simulink model "simulatore_motore"  (Simulink 8.3)
settings: Solver=ode45  StartTime=0.0  StopTime=30  RelTol=1e-3
values from neighbouring files (symbols this model uses):
  Beta = 17.7e-6    (= 1.77e-05)    [es1.m]
  J = 19.74e-6    (= 1.974e-05)    [es1.m]
  Km = 0.0535    [es1.m]
  Kpwm = 2.925    [es1.m]
  Kt = 0.02    [es1.m]
  La = 3.24e-3    (= 0.00324)    [es1.m]
  Ra = 6    [es1.m]
  Rs = 7.525    [es1.m]
  s = tf('s')    [es1.m]
  tau_a = 0.001    [es1.m]
  Td = -1e-4    (= -0.0001)    [es1.m]
libraries: cstblocks x8
settings Model: Creator=Indri  LastModifiedBy=HP  ExtModeTrigMode=oneshot  ExtModeArmWhenConnect=off
settings DataIOCC: LimitDataPoints=off
settings OptimizationCC: BlockReduction=off  BooleanDataType=off  ExpressionDepthLimit=2147483647  InitFltsAndDblsToZero=on
settings DebuggingCC: SaveWithParameterizedLinksMsg=none  SignalResolutionControl=TryResolveAllWithWarning  SolverPrmCheckMsg=none  MultiTaskDSMMsg=warning  MultiTaskCondExecSysMsg=none  FcnCallInpInsideContextMsg=UseLocalSettings
settings HardwareCC: TargetUnknown=on
settings RTWCC: IncludeERTFirstTime=on
settings GRTTargetCC: TargetFcnLib=ansi_tfl_tmw.mat

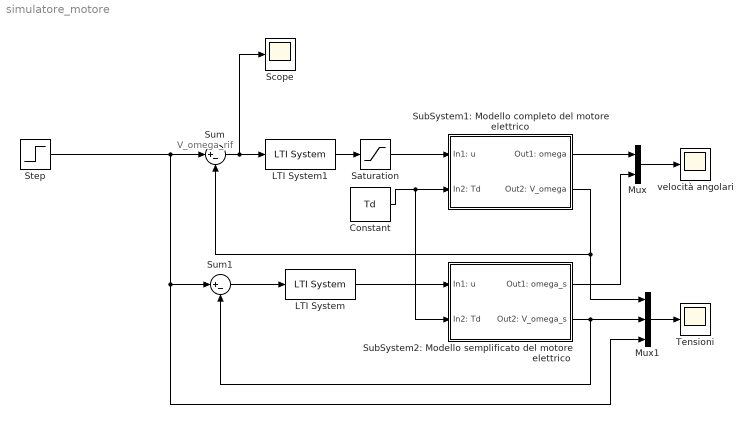
== system simulatore_motore ==
  note: V_omega_rif
  Constant : Constant  Value=Td
  LTI System : cstblocks/LTI System  sys=Cd  IC=[]
  LTI System1 : cstblocks/LTI System  sys=Cd  IC=[]
  Mux : Mux  Inputs=2
  Mux1 : Mux  Inputs=3
  Saturation : Saturate  UpperLimit=5  LowerLimit=-5
  Scope : Scope
      settings: MaxDataPoints=50000
  Step : Step  SampleTime=0
  SubSystem1: Modello completo del motore elettrico : Subsystem
  SubSystem2: Modello semplificato del motore elettrico : Subsystem
  Sum : Sum  Inputs=|+-  SaturateOnIntegerOverflow=on  InputSameDT=on  OutDataTypeStr=Inherit: Same as first input
  Sum1 : Sum  Inputs=|+-  SaturateOnIntegerOverflow=on  InputSameDT=on  OutDataTypeStr=Inherit: Same as first input
  Tensioni : Scope
      settings: YMin=-0.05  YMax=1
  velocità angolari : Scope
      settings: YMin=-2.5  YMax=50
  wires:
  SubSystem2: Modello semplificato del motore elettrico/1(Out1: omega_s) -> Mux/2
  SubSystem1: Modello completo del motore elettrico/1(Out1: omega) -> Mux/1
  Mux/1 -> velocità angolari/1
  Step/1 -> Sum/1, Sum1/1, Mux1/3
  Constant/1 -> SubSystem1: Modello completo del motore elettrico/2(In2: Td), SubSystem2: Modello semplificato del motore elettrico/2(In2: Td)
  SubSystem2: Modello semplificato del motore elettrico/2(Out2: V_omega_s) -> Sum1/2, Mux1/2
  Mux1/1 -> Tensioni/1
  SubSystem1: Modello completo del motore elettrico/2(Out2: V_omega) -> Sum/2, Mux1/1
  Sum1/1 -> LTI System/1
  LTI System/1 -> SubSystem2: Modello semplificato del motore elettrico/1(In1: u)
  Sum/1 -> Scope/1, LTI System1/1
  LTI System1/1 -> Saturation/1
  Saturation/1 -> SubSystem1: Modello completo del motore elettrico/1(In1: u)

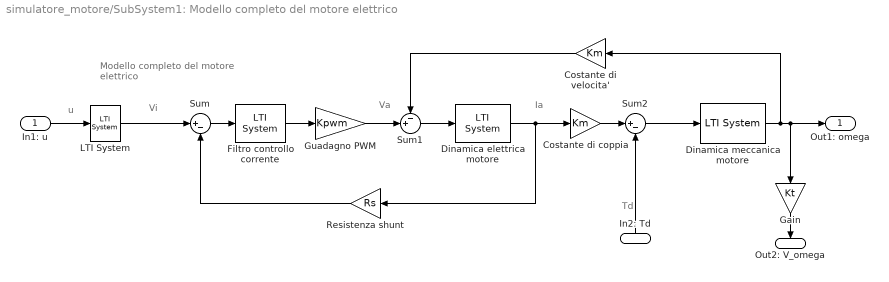
== system simulatore_motore/SubSystem1: Modello completo del motore elettrico ==
  note: Vi
  note: Ia
  note: Va
  note: u
  note: Td
  note: Modello completo
      | del motore elettrico
  In1: u : Inport
  In2: Td : Inport  Port=2
  Costante di coppia : Gain  Gain=Km  SaturateOnIntegerOverflow=on  OutDataTypeStr=Inherit: Same as input  ParamDataTypeStr=Inherit: Same as input
  Costante di velocita' : Gain  Gain=Km  SaturateOnIntegerOverflow=on  OutDataTypeStr=Inherit: Same as input  ParamDataTypeStr=Inherit: Same as input
  Dinamica elettrica motore : cstblocks/LTI System  sys=1/(Ra+s*La)  IC=[]
  Dinamica meccanica motore : cstblocks/LTI System  sys=1/(Beta+s*J)  IC=[]
  Filtro controllo corrente : cstblocks/LTI System  sys=1/(tau_a*s)  IC=[]
  Gain : Gain  Gain=Kt  SaturateOnIntegerOverflow=on  OutDataTypeStr=Inherit: Same as input  ParamDataTypeStr=Inherit: Same as input
  Guadagno PWM : Gain  Gain=Kpwm  SaturateOnIntegerOverflow=on  OutDataTypeStr=Inherit: Same as input  ParamDataTypeStr=Inherit: Same as input
  LTI System : cstblocks/LTI System  sys=1/s  IC=[]
  Resistenza shunt : Gain  Gain=Rs  SaturateOnIntegerOverflow=on  OutDataTypeStr=Inherit: Same as input  ParamDataTypeStr=Inherit: Same as input
  Sum : Sum  Inputs=|+-  SaturateOnIntegerOverflow=on  InputSameDT=on  OutDataTypeStr=Inherit: Same as first input
  Sum1 : Sum  Inputs=-+|  SaturateOnIntegerOverflow=on  InputSameDT=on  OutDataTypeStr=Inherit: Same as first input
  Sum2 : Sum  Inputs=|+-  SaturateOnIntegerOverflow=on  InputSameDT=on  OutDataTypeStr=Inherit: Same as first input
  Out1: omega : Outport
  Out2: V_omega : Outport  Port=2
  wires:
  Filtro controllo corrente/1 -> Guadagno PWM/1
  Guadagno PWM/1 -> Sum1/2
  Dinamica elettrica motore/1 -> Costante di coppia/1, Resistenza shunt/1
  Resistenza shunt/1 -> Sum/2
  Costante di coppia/1 -> Sum2/1
  Costante di velocita'/1 -> Sum1/1
  Sum/1 -> Filtro controllo corrente/1
  Sum1/1 -> Dinamica elettrica motore/1
  Sum2/1 -> Dinamica meccanica motore/1
  Dinamica meccanica motore/1 -> Costante di velocita'/1, Out1: omega/1, Gain/1
  In1: u/1 -> LTI System/1
  LTI System/1 -> Sum/1
  In2: Td/1 -> Sum2/2
  Gain/1 -> Out2: V_omega/1

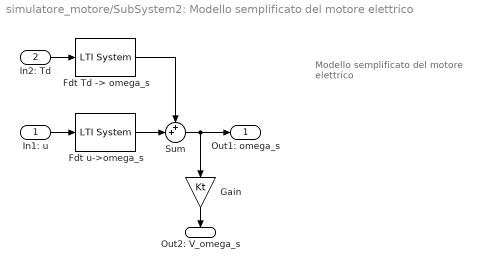
== system simulatore_motore/SubSystem2: Modello semplificato del motore elettrico ==
  note: Modello semplificato
      | del motore elettrico
  In1: u : Inport
  In2: Td : Inport  Port=2
  "Fdt Td -> omega_s" : cstblocks/LTI System  sys=Fd  IC=[]
  Fdt u->omega_s : cstblocks/LTI System  sys=F  IC=[]
  Gain : Gain  Gain=Kt  SaturateOnIntegerOverflow=on  OutDataTypeStr=Inherit: Same as input  ParamDataTypeStr=Inherit: Same as input
  Sum : Sum  Inputs=++|  SaturateOnIntegerOverflow=on  InputSameDT=on  OutDataTypeStr=Inherit: Same as first input
  Out1: omega_s : Outport
  Out2: V_omega_s : Outport  Port=2
  wires:
  In1: u/1 -> Fdt u->omega_s/1
  Fdt u->omega_s/1 -> Sum/2
  "Fdt Td -> omega_s"/1 -> Sum/1
  In2: Td/1 -> "Fdt Td -> omega_s"/1
  Sum/1 -> Out1: omega_s/1, Gain/1
  Gain/1 -> Out2: V_omega_s/1
